simulink model "DFIG_FILTER"  (R2023a)
settings: Solver=ode23t  StartTime=0.0  StopTime=25  MaxStep=1e-6  RelTol=1e-3
model workspace (MAT data in the model file):
  Ts_phasor = 10
undefined symbols (not defined in the file): Base_Power, D1, Delta, F, find_system, Fnom, gcbh, H, ILd_init, ILq_init, Imax_grid_conv, Init, j, Ki_dc_reg, Ki_grid_side_cur_reg, Ki_power_reg, Ki_Q, Ki_rotor_side_cur_reg, Ki_volt_reg, Kp_dc_reg, Kp_grid_side_cur_reg, Kp_power_reg, Kp_Q, Kp_rotor_side_cur_reg, Kp_volt_reg, L_RL, Llr, Lls, p, Pnom, power_A, power_B, power_D, R_RL, Rr, Rs, speed_A, speed_B, speed_C, speed_D, sps_rtmsupport, Vcontrol, Vnom, Wind_On
libraries: spsPower3phPhasorLib x9, spsOnDelayLib x9, spsThreePhaseVIMeasurementLib x8, simulink_extras x5, spsRMSLib x4, spsControlledCurrentSourceLib x4, spsGroundLib x3, spsSeriesRLCBranchLib x2, spsThreePhaseSeriesRLCBranchLib x2, spspowerguiLib x2, spsThreePhasePISectionLineLib x2, spsThreePhaseTransformerTwoWindingsLib x2
(part 1 of 6)
settings Model: Creator=Production  LastModifiedBy=Adham
settings SolverCC: ZeroCrossAlgorithm=Adaptive
settings DebuggingCC: IgnoredZcDiagnostic=none

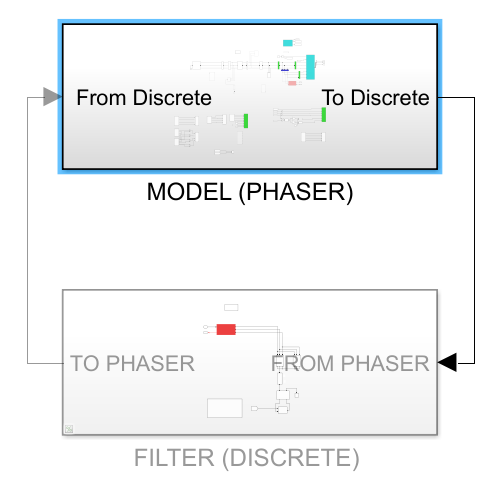
[thumbnail: Simulink's stored preview of the top-level diagram]
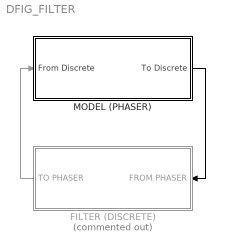
== system DFIG_FILTER ==
  "FILTER (DISCRETE) " : Subsystem  Commented=on
  MODEL (PHASER) : Subsystem
  wires:
  "FILTER (DISCRETE) "/1(TO PHASER) -> MODEL (PHASER)/1(" From Discrete")
  MODEL (PHASER)/1(To Discrete) -> "FILTER (DISCRETE) "/1(FROM PHASER)

== system DFIG_FILTER/FILTER (DISCRETE)  ==
  note: Rf
  note: Lf
  FROM PHASER : Inport
  " 1" : spsSeriesRLCBranchLib/Series RLC Branch  LConnTagsString=__new0  RConnTagsString=__new0  BranchType=RL  Resistance=0.15  Inductance=3e-3  SetiL0=off  InitialCurrent=0  Capacitance=1e-6  Setx0=off  InitialVoltage=0  Measurements=None
  CF : spsThreePhaseSeriesRLCBranchLib/Three-Phase Series RLC Branch  LConnTagsString=A|B|C  RConnTagsString=A|B|C  BranchType=C  Resistance=1  Inductance=1e-3  Capacitance=275e-6  Measurements=None
  D : spsUniversalBridgeLib/Universal Bridge  Arms=2  SnubberResistance=1e5  SnubberCapacitance=inf  Device=Diodes  Ron=10e-3  Lon=0  ForwardVoltages="[  0  0  ]"  ForwardVoltage=0  GTOparameters=[ 10e-6 , 20e-6 ]  IGBTparameters=[ 1e-6 , 2e-6 ]  Measurements=None  Measurements_2=None  converterType=Rectifier
  Discrete-to-Phasor Interface1 : spsDiscreteToPhasorInterfaceLib/Discrete-to-Phasor Interface  Rc=100  F=60  Ts_phasor=50e-6
      settings: LibrarySourceBlock=sps_lib/Utilities/Discrete-to-Phasor Interface
  Ground2 : spsGroundLib/Ground  LConnTagsString=a
  IGBT Switch Sa : spsIdealSwitchLib/Ideal Switch  Ron=0.001  Lon=0  IC=0  Rs=1e5  Cs=inf  Measurements=off
  RD : spsThreePhaseSeriesRLCBranchLib/Three-Phase Series RLC Branch  LConnTagsString=A|B|C  RConnTagsString=A|B|C  BranchType=R  Resistance=1e6  Inductance=23e-3  Capacitance=1e-6  Measurements=None
  controller1 : Subsystem
  powergui : spspowerguiLib/powergui  Priority=1  SimulationMode=Discrete  SampleTime=50e-6  frequency=60  Iterations=50  frequencyindice=0  Pbase=100e6  ErrMax=1e-4  UnitsV=kV  UnitsW=MW  buscounter=0  FunctionMessages=off  echomessages=off  EnableUseOfTLC=off  CurrentSourceSwitches=off  DisableSnubberDevices=off  DisableRonSwitches=off  DisableVfSwitches=off  DisplayEquations=off  AutomaticDiscreteSolvers=off  SolverType=Tustin/Backward Euler (TBE)  Interpol=off  ExternalGateDelay=off  methode=off  Ts=100  x0status=blocks  SPID=on  SwTol=0  HookPort=off  NonlinearTolerance=1e-4  nMaxIteration=100  ContinueOnMaxIteration=off  RestoreLinks=warning  ResistiveCurrentMeasurement=off  Frange=[0:2:500]  Ylog=off  Xlog=on  ShowGrid=off  save=off  variable=ZData  structure=0  ZoomFFT=off  StartTime=0.0  cycles=1  DisplayStyle=1  fundamental=60  FreqAxis=off  MaxFrequency=1000  frequencyindicesteady=1  RmsSteady=1  display=off
  TO PHASER : Outport
  wires:
  Discrete-to-Phasor Interface1/1 -> TO PHASER/1
  FROM PHASER/1 -> Discrete-to-Phasor Interface1/1
  [Sa] -> IGBT Switch Sa/1
  connections:
  RD/LConn3 -- Discrete-to-Phasor Interface1/LConn3 -- CF/LConn3
  RD/RConn1 -- CF/RConn3 -- CF/RConn1 -- RD/RConn3 -- RD/RConn2
  CF/RConn2 -- " 1"/LConn1
  IGBT Switch Sa/RConn1 -- D/RConn2
  " 1"/RConn1 -- D/LConn1
  IGBT Switch Sa/LConn1 -- D/RConn1
  D/LConn2 -- Ground2/LConn1
  RD/LConn2 -- Discrete-to-Phasor Interface1/LConn2 -- CF/LConn2
  CF/LConn1 -- Discrete-to-Phasor Interface1/LConn1 -- RD/LConn1

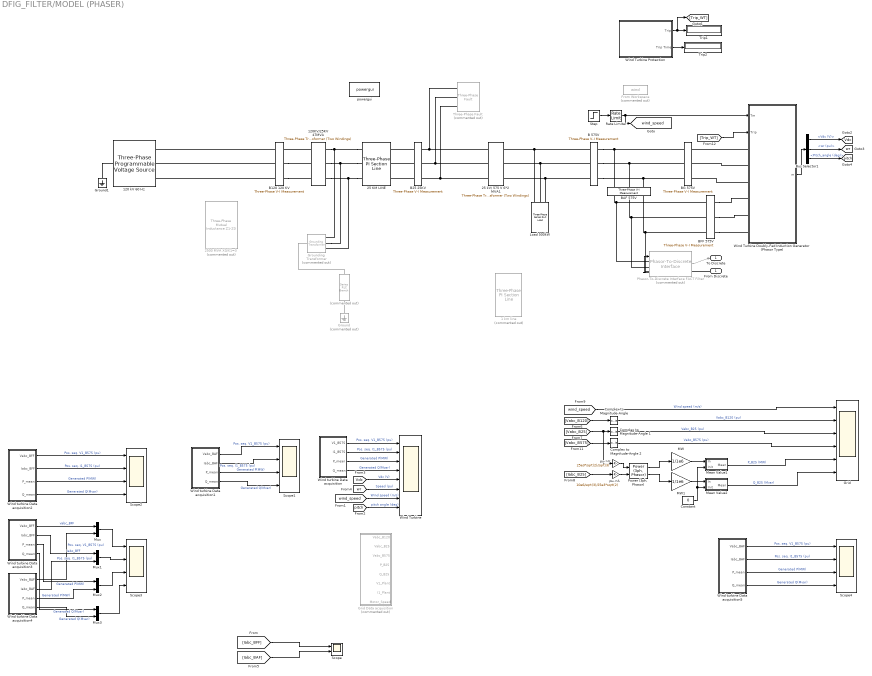
== system DFIG_FILTER/MODEL (PHASER) ==
  " From Discrete" : Inport
  " " : spsSeriesRLCBranchLib/Series RLC Branch  Commented=on  LConnTagsString=__new0  RConnTagsString=__new0  BranchType=R  Resistance=3.3  Inductance=0.003  SetiL0=off  InitialCurrent=0  Capacitance=1e-6  Setx0=off  InitialVoltage=0  Measurements=Branch voltage and current
  1 km line : spsThreePhasePISectionLineLib/Three-Phase PI Section Line  Commented=on  LConnTagsString=a|b|c  RConnTagsString=A|B|C  Length=1  Frequency=60  Resistances=[0.1153 0.413]  Inductances=[1.05e-3 3.32e-3]  Capacitances=[11.33e-009 5.01e-009]
  120 kV 60 Hz : spsThreePhaseProgrammableVoltageSourceLib/Three-Phase Programmable Voltage Source  PositiveSequence=[120e3 0 60]  VariationEntity=None  VariationType=Table of time-amplitude pairs  VariationTypeAlt=Step  VariationStep=0.5  VariationRate=10  VariationMagnitude=0.3  VariationFrequency=2  VariationTiming=[1 2]  VariationPhaseA=off  Amplitudes=[1 0.8 1.2 1.0]  TimeValues=[0 0.1 0.15 0.2]  HarmonicGeneration=off  HarmonicA=[3 0.2 -25 0]  HarmonicB=[2 0.15 35 2]  Timing="[0.05  3]"  BusType=swing  Pref=0  Qref=0  Qmin=-inf  Qmax=inf
  120KV/25KV 47MVA : spsThreePhaseTransformerTwoWindingsLib/Three-Phase Transformer (Two Windings)  Winding1Connection=Yg  Winding2Connection=Delta (D1)  CoreType=Three single-phase transformers  SetSaturation=off  Hysteresis=off  DataFile='hysteresis'  SetInitialFlux=off  Measurements=None  UNITS=pu  NominalPower=[47e6 60 ]  Winding1="[ 120e3  0.08/30   0.08 ]"  Winding2="[ 25e3  0.08/30  0.08]"  Rm=500/((120e3)^2/(Base_Power))  Lm=500/((120e3)^2/(Base_Power))  L0=0.5  Saturation=[ 0,0 ; 0.0024,1.2 ; 1.0,1.52 ]  InitialFluxes=[ 0.8 , -0.8 , 0.7 ]  BreakLoop=off  DiscreteSolver=Trapezoidal iterative  DataType=off  TransfoNumber=1
  25 KM LINE : spsThreePhasePISectionLineLib/Three-Phase PI Section Line  LConnTagsString=a|b|c  RConnTagsString=A|B|C  Length=25  Frequency=60  Resistances=[0.1153 0.413]  Inductances=[1.05e-3 3.32e-3]  Capacitances=[11.33e-009 5.01e-009]
  25 kV/ 575 V 6*2 MVA1 : spsThreePhaseTransformerTwoWindingsLib/Three-Phase Transformer (Two Windings)  Winding1Connection=Yg  Winding2Connection=Delta (D1)  CoreType=Three single-phase transformers  SetSaturation=off  Hysteresis=off  DataFile='hysteresis'  SetInitialFlux=off  Measurements=None  UNITS=pu  NominalPower="[2e6*6  60]"  Winding1=[25e3 , 0.025/30 , 0.025]  Winding2=[575, 0.025/30 , 0.025]  Rm=500/((25e3)^2/(Base_Power))  Lm=500/((25e3)^2/(Base_Power))  L0=0.5  Saturation=[ 0,0 ; 0.0024,1.2 ; 1.0,1.52 ]  InitialFluxes=[ 0.8 , -0.8 , 0.7 ]  BreakLoop=off  DiscreteSolver=Trapezoidal iterative  DataType=off  TransfoNumber=0
  2500 MVA X0/X1=3 : spsThreePhaseMutualInductanceZ1Z0Lib/Three-Phase Mutual Inductance Z1-Z0  Commented=on  LConnTagsString=a|b|c  RConnTagsString=A|B|C  PositiveSequence="[0.1  1.0/(2*pi*60)] *120e3^2/2500e6"  ZeroSequence="[0.3  3.0/(2*pi*60)] *120e3^2/2500e6"
      settings: AttributesFormatString=\n
      settings: LibrarySourceBlock=|
      | sps_lib/Power Grid Elements/Three-Phase
      | Mutual Inductance
      | Z1-Z0
  B 575V : spsThreePhaseVIMeasurementLib/Three-Phase V-I Measurement  VoltageMeasurement=phase-to-ground  SetLabelV=on  LabelV=Vabc_B575  Vpu=on  VpuLL=off  CurrentMeasurement=yes  SetLabelI=on  LabelI=Iabc_BL  Ipu=on  Pbase=Base_Power  Vbase=575  OutputType=Magnitude  PhasorSimulation=on  PSBequivalent=0
  B120 120 KV : spsThreePhaseVIMeasurementLib/Three-Phase V-I Measurement  VoltageMeasurement=phase-to-ground  SetLabelV=on  LabelV=Vabc_B120  Vpu=on  VpuLL=off  CurrentMeasurement=no  SetLabelI=on  LabelI=Iabc  Ipu=on  Pbase=100e6  Vbase=120e3  OutputType=Complex  PhasorSimulation=on  PSBequivalent=0
  B25 25KV : spsThreePhaseVIMeasurementLib/Three-Phase V-I Measurement  VoltageMeasurement=phase-to-ground  SetLabelV=on  LabelV=Vabc_B25  Vpu=on  VpuLL=off  CurrentMeasurement=yes  SetLabelI=on  LabelI=Iabc_B25  Ipu=on  Pbase=Base_Power  Vbase=25e3  OutputType=Complex  PhasorSimulation=on  PSBequivalent=0
  BAF 575V : spsThreePhaseVIMeasurementLib/Three-Phase V-I Measurement  VoltageMeasurement=phase-to-ground  SetLabelV=on  LabelV=Vabc_BAF  Vpu=on  VpuLL=off  CurrentMeasurement=yes  SetLabelI=on  LabelI=Iabc_BAF  Ipu=on  Pbase=100e6  Vbase=575  OutputType=Magnitude  PhasorSimulation=on  PSBequivalent=0
  BFF 575V : spsThreePhaseVIMeasurementLib/Three-Phase V-I Measurement  VoltageMeasurement=phase-to-ground  SetLabelV=on  LabelV=Vabc_BFF  Vpu=on  VpuLL=off  CurrentMeasurement=yes  SetLabelI=on  LabelI=Iabc_BFF  Ipu=on  Pbase=Base_Power  Vbase=575  OutputType=Magnitude  PhasorSimulation=on  PSBequivalent=0
  "BG 575V " : spsThreePhaseVIMeasurementLib/Three-Phase V-I Measurement  VoltageMeasurement=phase-to-ground  SetLabelV=on  LabelV=Vabc_BG  Vpu=on  VpuLL=off  CurrentMeasurement=yes  SetLabelI=on  LabelI=Iabc_BG  Ipu=on  Pbase=Base_Power  Vbase=575  OutputType=Complex  PhasorSimulation=on  PSBequivalent=0
  Bus Selector1 : BusSelector  OutputSignals=Vdc (V),wr (pu),Pitch_angle (deg)
  "Complex to Magnitude-Angle " : ComplexToMagnitudeAngle  Output=Magnitude
  Complex to Magnitude-Angle 1 : ComplexToMagnitudeAngle  Output=Magnitude
  Complex to Magnitude-Angle 2 : ComplexToMagnitudeAngle  Output=Magnitude
  Constant : Constant  Value=0
  From Workspace : FromWorkspace  Commented=on  VariableName=wind
  Grid : Scope  NumInputPorts=6
  Grid Data acquisition : Subsystem  Commented=on
  Ground : spsGroundLib/Ground  Commented=on  LConnTagsString=a
  Ground1 : spsGroundLib/Ground  LConnTagsString=a
  "Grounding Transformer " : spsGroundingTransformerLib/Grounding Transformer   Commented=on  UNITS=pu  NominalPower="[100e6   60]"  NominalVoltage=25e3  ZeroSequenceImpedance_pu=[0.025 0.75]  MagnetizationBranch_pu=[500 500]  ZeroSequenceImpedance_SI=[0.052083 589.05]  MagnetizationBranch_SI=[1041.7 3.927e+005]  Measurements=None
  Load 500kW : spsThreePhaseSeriesRLCLoadLib/Three-Phase Series RLC Load  LConnTagsString=A|B|C  Configuration=Y (grounded)  NominalVoltage=575  Vabc=[1e3 1e3 1e3]  Vabcp=[1e3 1e3 1e3]  NominalFrequency=60  UnbalancedPower=off  ActivePower=500e3  InductivePower=0  CapacitivePower=0  Pabc=[10e3 9e3 11e3]  QLabc=[100 90 110]  QCabc=[100 90 110]  Pabcp=[10e3 9e3 11e3]  QLabcp=[100 90 110]  QCabcp=[100 90 110]  Measurements=None  LoadType=constant Z
  MW : Gain  Gain=1/1e6  SaturateOnIntegerOverflow=on  OutDataTypeStr=Inherit: Same as input  ParamDataTypeStr=Inherit: Same as input
  MW1 : Gain  Gain=1/1e6  SaturateOnIntegerOverflow=on  OutDataTypeStr=Inherit: Same as input  ParamDataTypeStr=Inherit: Same as input
  Mean Value1 : Subsystem  mask(Mean value){Period=1/60}
      mask prompts: Period "Averaging period (s):"
      mask help: This block uses the running window averaging technique to compute the mean value of the input signal over the specified period.
  Mean Value2 : Subsystem  mask(Mean value){Period=1/60}
      mask prompts: Period "Averaging period (s):"
      mask help: This block uses the running window averaging technique to compute the mean value of the input signal over the specified period.
  Mux{,1..3} (4 alike) : Mux  Inputs=2
  Phasor-To-Discrete Interface FACT Filter : spsPhasorToDiscreteInterfaceLib/Phasor-To-Discrete Interface  Commented=on  Rc=100  F=60  Ts=50e-6
      settings: LibrarySourceBlock=sps_lib/Utilities/Phasor-To-Discrete Interface
  "Power (3ph, Phasor)" : spsPower3phPhasorLib/Power (3ph, Phasor)
  Rate Limiter : RateLimiter
  Scope : Scope  NumInputPorts=2
  Scope{1..4} (4 alike) : Scope  NumInputPorts=4
  Step : Step  Time=2  Before=4  After=14  SampleTime=0
  Three-Phase Fault : spsThreePhaseFaultLib/Three-Phase Fault  Commented=on  InitialStates=0  FaultA=on  FaultB=off  FaultC=off  GroundFault=on  SwitchTimes="[1/60  5/60]"  External=off  SwitchStatus=NaN  FaultResistance=0.001  GroundResistance=0.01  SnubberResistance=1e4  SnubberCapacitance=inf  Measurements=None
  Trip1 : Display
  Trip2 : Display
  Wind Turbine : Scope  NumInputPorts=8
  Wind Turbine Doubly-Fed Induction Generator (Phasor Type) : Subsystem  AncestorBlock=|  DialogController=POWERSYS.PowerSysDialog  LoadFcn=sps_rtmsupport('LoadFcn',gcbh); %find_system(gcs,'FollowLinks', 'on', 'LookUnderMasks', 'all');  StartFcn=sps_rtmsupport('StartFcn',gcbh);  StopFcn=sps_rtmsupport('StopFcn',gcbh);  mask(Wind Turbine Doubly-Fed Induction Generator (Phasor Type)){ExternalTm=off, nom=[1.5e6/0.9 575 60], sta=[ 0.00706 0.171], rot=[ 0.005 0.156], Lm=2.90, mec=[5.04 0.01 3], init=[0.2 0 0 0 0 0], speed_power=[0 0; 0.24 0.007; 0.36 0.024; 0.6 0.112; 0.96 0.46; 1.2 0.898; 1.5 0.898], Pmec=1.5e6, speed_ABCD=[0.7 0.71 1.2 1.21], power_C=0.73, wind_point_C=12, pitch_gain=500, pitch_max=45, pitch_rate=2, Pmax=0.5, Lchoke=[0.15 0.15/100], init_inductor=[0 90], Vdc_nom=1200, capacitor=10000e-6, ControlVQ=Voltage regulation, Vref=1.0, ExternalVref=off, Qref=0, ExternalQref=on, Iq_ref=0, ExternalIqref=off, Kpi_volt_reg=[1.25 300], Xs=0.02, Kpi_Q=[0.05 5], Kpi_power_reg=[1 100], Kpi_dc_reg=[0.002 0.05], Kpi_grid_side_cur_reg=[1 100], Kpi_rotor_side_cur_reg=[0.3 8], V_slew_rate=100, Q_slew_rate=100, power_slew_rate=1, current_slew_rate=200}
      | sps_lib/Electrical Machines/Wind Turbine
      | Doubly-Fed Induction Generator
      | (Phasor Type)
      mask prompts: ExternalTm "External turbine (Tm mechanical torque input)"; nom "Nominal power, line-to-line voltage, frequency [Pn(VA), Vn(Vrms), fn(Hz)]:"; sta "Stator [Rs, Lls] (pu):"; rot "Rotor [Rr', Llr' ] (pu):"; Lm "Magnetizing inductance Lm (pu):"; mec "Inertia constant, friction factor, and pairs of poles [H(s), F(pu),  p ]:"; init "Initial conditions [s,  th(deg),  Is(pu), ph_Is(deg),  Ir(pu),  ph_Ir(deg)]:"; speed_power "Electric power-speed characteristic: [wr1(pu) p1(pu); wr2(pu) p2(pu); ... ]"; Pmec "Nominal wind turbine mechanical output power (W):"; speed_ABCD "Tracking characteristic speeds: [speed_A(pu) ... speed_D(pu)]"; power_C "Power at point C (pu/mechanical power):"; wind_point_C "Wind speed at point C (m/s):"; pitch_gain "Pitch angle controller gain [Kp]:"; pitch_max "Maximum pitch angle (deg):"; pitch_rate "Maximum rate of change of pitch angle (deg/s):"; Pmax "Converter maximum power (pu):"; Lchoke "Grid-side coupling inductor [L (pu) R (pu)]:"; init_inductor "Coupling inductor initial current: [ IL(pu) ph_IL(deg)]"; Vdc_nom "Nominal DC bus voltage (V):"; capacitor "DC bus capacitor (F):"; ControlVQ "Mode:"; Vref "Reference grid voltage Vref (pu):"; ExternalVref "External"; Qref "Generated reactive power Qref (pu):"; ExternalQref "External"; Iq_ref "Grid-side converter generated reactive current reference (Iq_ref) (pu):"; ExternalIqref "External"; Kpi_volt_reg "Grid voltage regulator gains: [Kp Ki]"; Xs "Droop Xs (pu):"; Kpi_Q "Reactive power regulator gains: [Kp Ki]"; Kpi_power_reg "Power regulator gains: [Kp Ki]"; Kpi_dc_reg "DC bus voltage regulator gains: [Kp Ki]"; Kpi_grid_side_cur_reg "Grid-side converter current regulator gains: [Kp Ki]"; Kpi_rotor_side_cur_reg "Rotor-side converter current regulator gains: [Kp Ki]"; V_slew_rate "Maximum rate of change of reference grid voltage (pu/s):"; Q_slew_rate "Maximum rate of change of reference reactive power (pu/s):"; power_slew_rate "Maximum rate of change of reference power (pu/s):"; current_slew_rate "Maximum rate of change of converter  reference currents (pu/s):"
      mask help: Implements a phasor model of a doubly-fed induction generator driven by a wind turbine.
      mask init:
      | [Pnom,Vnom,Fnom,Rs,Lls,Rr,Llr,H,p,F,Wind_On,FACTSroot,mag_IL_init,ph_IL_init,ILd_init,ILq_init,Imax_grid_conv,speed_A,speed_B,speed_C,speed_D,power_A,power_B,power_D,L_RL,R_RL,Kp_volt_reg,Ki_volt_reg,Kp_Q,Ki_Q,Kp_power_reg,Ki_power_reg,Kp_dc_reg,Ki_dc_reg,Kp_grid_side_cur_reg,Ki_grid_side_cur_reg,Kp_rotor_side_cur_reg,Ki_rotor_side_cur_reg,Vcontrol] ...
      |     = WindTurbineInit (nom,sta,rot,mec,ExternalTm,1,gcbh,Pmax,Lchoke,init_inductor,speed_ABCD,power_C,Kpi_volt_reg,Kpi_Q,Kpi_power_reg,Kpi_dc_reg,Kpi_grid_side_cur_reg,Kpi_rotor_side_cur_reg,ControlVQ);
      settings: CopyFcn=sps_rtmsupport('CopyFcn',gcbh);  DeleteFcn=sps_rtmsupport('DeleteFcn',gcbh);  UndoDeleteFcn=sps_rtmsupport('UndoDeleteFcn',gcbh);  ModelCloseFcn=sps_rtmsupport('ModelCloseFcn',gcbh);  PreSaveFcn=sps_rtmsupport('PreSaveFcn',gcbh);  PostSaveFcn=sps_rtmsupport('PostSaveFcn',gcbh);  NameChangeFcn=sps_rtmsupport('NameChangeFcn',gcbh);  PreCopyFcn=sps_rtmsupport('PreCopyFcn',gcbh);  OpenFcn=sps_rtmsupport('OpenFcn',gcbh, [1 21,23,25,27]);  CloseFcn=sps_rtmsupport('CloseFcn',gcbh);  PreDeleteFcn=sps_rtmsupport('PreDeleteFcn',gcbh);
      settings: LibrarySourceBlock=|
      | sps_lib/Electrical Machines/Wind Turbine
      | Doubly-Fed Induction Generator
      | (Phasor Type)
      mask Help: helpview(psbhelp)
      mask Callback ExternalTm: WindTurbineCback(gcbh);
      mask TypeOptions ControlVQ: Voltage regulation | Var regulation
      mask Callback ControlVQ: WindTurbineCback(gcbh);
      mask Callback ExternalVref: WindTurbineCback(gcbh);
      mask Callback ExternalQref: WindTurbineCback(gcbh);
      mask Callback ExternalIqref: WindTurbineCback(gcbh);
      mask DialogControl generatordata Prompt: Generator
      mask DialogControl turbinedata Prompt: Turbine
      mask DialogControl Display Prompt: Display wind turbine power characteristics
      mask DialogControl Display Callback: WindTurbineDisplay(gcbh);
      mask DialogControl convertersdata Prompt: Converters
      mask DialogControl controlparameters Prompt: Control
      mask Display:
      | port_label('LConn',1,'A_stator')
      | port_label('LConn',2,'B_stator')
      | port_label('LConn',3,'C_stator')
      | port_label('LConn',4,'A_rotor')
      | port_label('LConn',5,'B_rotor')
      | port_label('LConn',6,'C_rotor')
      | 
      | port_label('output',1,'m')
      | 
      | Block = gcbh;
      | switch get_param(Block,'ExternalTm')
      |     case 'on'
      |         port_label('input',1,'Tm')
      |     case 'off'
      |         port_label('input',1,'wind')
      | end
      | 
      | x = 2;
      | 
      | switch get_param(Block,'ControlVQ')
      |     case 'Voltage regulation'
      |         switch get_param(Block,'ExternalVref')
      |             case 'on'
      |                 port_label('input',2,'Vref');
      |                 x = 3;
      |         end
      |     case 'Var regulation'
      |         switch get_param(Block,'ExternalQref')
      |             case 'on'
      |                 port_label('input',2,'Qref');
      |                 x = 3;
      |         end
      | end
      | 
      | switch get_param(Block,'ExternalIqref')
      |     case 'on'
      |         port_label('input',x,'Iq_ref');
      |         x = x +1;
      | end
      | 
      | port_label('input',x,'trip');
  Wind Turbine Protection : Subsystem
      mask Display: disp('Wind\nTurbine\nProtection')
  Wind turbine Data acquisition : Subsystem
  Wind turbine Data acquisition1 : Subsystem
  Wind turbine Data acquisition2 : Subsystem
  Wind turbine Data acquisition3 : Subsystem
  Wind turbine Data acquisition4 : Subsystem
  Wind turbine Data acquisition5 : Subsystem
  powergui : spspowerguiLib/powergui  Priority=1  SimulationMode=Discrete phasor  SampleTime=5e-6  frequency=60  Iterations=50  frequencyindice=60  Pbase=100e6  ErrMax=1e-4  UnitsV=kV  UnitsW=MW  buscounter=0  FunctionMessages=off  echomessages=off  EnableUseOfTLC=off  CurrentSourceSwitches=off  DisableSnubberDevices=off  DisableRonSwitches=off  DisableVfSwitches=off  DisplayEquations=off  AutomaticDiscreteSolvers=off  SolverType=Tustin/Backward Euler (TBE)  Interpol=off  ExternalGateDelay=off  methode=off  Ts=100  x0status=blocks  SPID=on  SwTol=0  HookPort=off  NonlinearTolerance=1e-4  nMaxIteration=100  ContinueOnMaxIteration=off  RestoreLinks=warning  ResistiveCurrentMeasurement=off  Frange=[0:2:500]  Ylog=off  Xlog=on  ShowGrid=off  save=off  variable=ZData  structure=0  ZoomFFT=off  StartTime=0.0  cycles=1  DisplayStyle=1  fundamental=60  FreqAxis=off  MaxFrequency=1000  frequencyindicesteady=1  RmsSteady=1  display=off
  pu->A : Gain  Gain=10e6/sqrt(3)/25e3*sqrt(2)  SaturateOnIntegerOverflow=on  OutDataTypeStr=Inherit: Same as input  ParamDataTypeStr=Inherit: Same as input
  pu->V : Gain  Gain=25e3*sqrt(2)/sqrt(3)  SaturateOnIntegerOverflow=on  OutDataTypeStr=Inherit: Same as input  ParamDataTypeStr=Inherit: Same as input
  To Discrete : Outport
  tag scope: Vdc=global, pitch=global, wind_speed=global, wr=global
  wires:
  [Trip_WT] -> Wind Turbine Doubly-Fed Induction Generator (Phasor Type)/2(Trip)
  Bus Selector1/3 -> [pitch]  "<Pitch_angle (deg)>"
  Bus Selector1/1 -> [Vdc]  "<Vdc (V)>"
  Wind Turbine Doubly-Fed Induction Generator (Phasor Type)/1(m) -> Bus Selector1/1
  " From Discrete"/1 -> Phasor-To-Discrete Interface FACT Filter/1
  Bus Selector1/2 -> [wr]  "<wr (pu)>"
  Phasor-To-Discrete Interface FACT Filter/1 -> To Discrete/1
  Wind turbine Data acquisition/4(Q_mean) -> Wind Turbine/4  "Generated Q(Mvar)"
  [wind_speed] -> Wind Turbine/7  "Wind speed (m/s)"
  Complex to Magnitude-Angle 2/1 -> Grid/4  "Vabc_B575 (pu)"
  Wind turbine Data acquisition/2(I1_B575) -> Wind Turbine/2  "Pos. seq. I1_B575 (pu)"
  Mean Value1/1(Mean) -> Grid/5  "P_B25 (MW)"
  Complex to Magnitude-Angle 1/1 -> Grid/3  "Vabc_B25 (pu)"
  [wr] -> Wind Turbine/6  "Speed (pu)"
  Wind turbine Data acquisition/3(P_mean) -> Wind Turbine/3  "Generated P(MW)"
  "Complex to Magnitude-Angle "/1 -> Grid/2  "Vabc_B120 (pu)"
  [pitch] -> Wind Turbine/8  "pitch angle (deg)"
  Mean Value2/1(Mean) -> Grid/6  "Q_B25 (Mvar)"
  Wind turbine Data acquisition/1(V1_B575) -> Wind Turbine/1  "Pos. seq. V1_B575 (pu)"
  [Vdc] -> Wind Turbine/5  "Vdc (V)"
  Wind Turbine Protection/2(Trip Time) -> Trip2/1
  Wind Turbine Protection/1(Trip) -> [Trip_WT], Trip1/1
  Step/1 -> Rate Limiter/1
  Rate Limiter/1 -> [wind_speed], Wind Turbine Doubly-Fed Induction Generator (Phasor Type)/1("Tm ")
  [Iabc_BFF] -> Scope/1
  [Iabc_BAF] -> Scope/2
  Wind turbine Data acquisition1/1(Vabc_BAF) -> Scope1/1  "Pos. seq. V1_B575 (pu)"
  Wind turbine Data acquisition1/2(Iabc_BAF) -> Scope1/2  "Pos. seq. I1_B575 (pu)"
  Wind turbine Data acquisition1/3(P_mean) -> Scope1/3  "Generated P(MW)"
  Wind turbine Data acquisition1/4(Q_mean) -> Scope1/4  "Generated Q(Mvar)"
  Wind turbine Data acquisition2/2(Iabc_BFF) -> Scope2/2  "Pos. seq. I1_B575 (pu)"
  Wind turbine Data acquisition2/3(P_mean) -> Scope2/3  "Generated P(MW)"
  Wind turbine Data acquisition2/1(Vabc_BFF) -> Scope2/1  "Pos. seq. V1_B575 (pu)"
  Wind turbine Data acquisition2/4(Q_mean) -> Scope2/4  "Generated Q(Mvar)"
  Wind turbine Data acquisition3/1(Vabc_BFF) -> Mux/1  "vabc_BFF"
  Wind turbine Data acquisition4/1(Vabc_BAF) -> Mux/2  "Pos. seq. V1_B575 (pu)"
  Wind turbine Data acquisition3/2(Iabc_BFF) -> Mux1/1  "Iabc_BFF"
  Wind turbine Data acquisition4/2(Iabc_BAF) -> Mux1/2  "Pos. seq. I1_B575 (pu)"
  Wind turbine Data acquisition3/3(P_mean) -> Mux2/1  "Generated P(MW)"
  Wind turbine Data acquisition4/3(P_mean) -> Mux2/2  "Generated P(MW)"
  Wind turbine Data acquisition4/4(Q_mean) -> Mux3/2  "Generated Q(Mvar)"
  Wind turbine Data acquisition3/4(Q_mean) -> Mux3/1  "Generated Q(Mvar)"
  Mux/1 -> Scope3/1
  Mux1/1 -> Scope3/2
  Mux2/1 -> Scope3/3
  Mux3/1 -> Scope3/4
  [Vabc_B575] -> Complex to Magnitude-Angle 2/1
  [Vabc_B120] -> "Complex to Magnitude-Angle "/1
  MW/1 -> Mean Value1/1(In)
  MW1/1 -> Mean Value2/1(In)
  "Power (3ph, Phasor)"/1 -> MW/1
  pu->A/1 -> "Power (3ph, Phasor)"/2
  "Power (3ph, Phasor)"/2 -> MW1/1
  Constant/1 -> Mean Value1/2(Init), Mean Value2/2(Init)
  pu->V/1 -> "Power (3ph, Phasor)"/1
  [Iabc_B25] -> pu->A/1
  [Vabc_B25] -> Complex to Magnitude-Angle 1/1, pu->V/1
  Wind turbine Data acquisition5/3(P_mean) -> Scope4/3  "Generated P(MW)"
  Wind turbine Data acquisition5/2(Iabc_BAF) -> Scope4/2  "Pos. seq. I1_B575 (pu)"
  Wind turbine Data acquisition5/4(Q_mean) -> Scope4/4  "Generated Q(Mvar)"
  Wind turbine Data acquisition5/1(Vabc_BAF) -> Scope4/1  "Pos. seq. V1_B575 (pu)"
  [wind_speed] -> Grid/1  "Wind speed (m/s)"
  connections:
  25 KM LINE/LConn1 -- "Grounding Transformer "/LConn1 -- 120KV/25KV 47MVA/RConn1
  B25 25KV/LConn3 -- 25 KM LINE/RConn3
  25 KM LINE/LConn3 -- "Grounding Transformer "/LConn3 -- 120KV/25KV 47MVA/RConn3
  B25 25KV/RConn1 -- 25 kV/ 575 V 6*2 MVA1/LConn1 -- Three-Phase Fault/LConn1
  " "/LConn1 -- "Grounding Transformer "/RConn1
  Load 500kW/LConn1 -- B 575V/LConn1 -- 25 kV/ 575 V 6*2 MVA1/RConn1
  Ground1/LConn1 -- 120 kV 60 Hz/LConn1
  B25 25KV/RConn3 -- 25 kV/ 575 V 6*2 MVA1/LConn3 -- Three-Phase Fault/LConn3
  25 KM LINE/LConn2 -- "Grounding Transformer "/LConn2 -- 120KV/25KV 47MVA/RConn2
  B120 120 KV/LConn3 -- 120 kV 60 Hz/RConn3
  B120 120 KV/LConn2 -- 120 kV 60 Hz/RConn2
  Ground/LConn1 -- " "/RConn1
  B25 25KV/RConn2 -- 25 kV/ 575 V 6*2 MVA1/LConn2 -- Three-Phase Fault/LConn2
  B25 25KV/LConn1 -- 25 KM LINE/RConn1
  120KV/25KV 47MVA/LConn1 -- B120 120 KV/RConn1
  B120 120 KV/LConn1 -- 120 kV 60 Hz/RConn1
  B25 25KV/LConn2 -- 25 KM LINE/RConn2
  B120 120 KV/RConn3 -- 120KV/25KV 47MVA/LConn3
  B120 120 KV/RConn2 -- 120KV/25KV 47MVA/LConn2
  Load 500kW/LConn2 -- B 575V/LConn2 -- 25 kV/ 575 V 6*2 MVA1/RConn2
  BFF 575V/RConn1 -- Wind Turbine Doubly-Fed Induction Generator (Phasor Type)/LConn4
  BFF 575V/RConn2 -- Wind Turbine Doubly-Fed Induction Generator (Phasor Type)/LConn5
  BFF 575V/RConn3 -- Wind Turbine Doubly-Fed Induction Generator (Phasor Type)/LConn6
  Load 500kW/LConn3 -- B 575V/LConn3 -- 25 kV/ 575 V 6*2 MVA1/RConn3
  BFF 575V/LConn1 -- Phasor-To-Discrete Interface FACT Filter/LConn1 -- BAF 575V/RConn1
  BFF 575V/LConn2 -- Phasor-To-Discrete Interface FACT Filter/LConn2 -- BAF 575V/RConn2
  BFF 575V/LConn3 -- BAF 575V/RConn3 -- Phasor-To-Discrete Interface FACT Filter/LConn3
  Wind Turbine Doubly-Fed Induction Generator (Phasor Type)/LConn1 -- "BG 575V "/RConn1
  Wind Turbine Doubly-Fed Induction Generator (Phasor Type)/LConn2 -- "BG 575V "/RConn2
  Wind Turbine Doubly-Fed Induction Generator (Phasor Type)/LConn3 -- "BG 575V "/RConn3
  "BG 575V "/LConn3 -- B 575V/RConn3 -- BAF 575V/LConn3
  "BG 575V "/LConn2 -- B 575V/RConn2 -- BAF 575V/LConn2
  "BG 575V "/LConn1 -- B 575V/RConn1 -- BAF 575V/LConn1

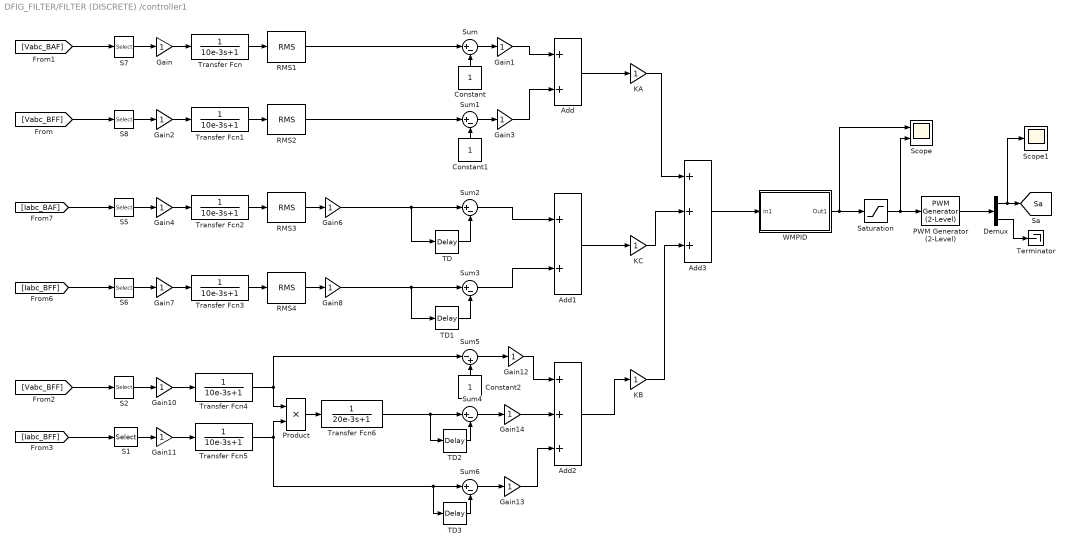
== system DFIG_FILTER/FILTER (DISCRETE) /controller1 ==
  Add : Sum
  Add1 : Sum
  Add2 : Sum  Inputs=+++
  Add3 : Sum  Inputs=+++
  Constant : Constant
  Constant1 : Constant
  Constant2 : Constant
  Demux : Demux  Outputs=2
  Gain{,1..4,6..8,10..14} (13 alike) : Gain
  KA : Gain
  KB : Gain
  KC : Gain
  PWM Generator (2-Level) : spsPWMGenerator2LevelLib/PWM Generator (2-Level)  ModulatorType=Three-phase bridge (6 pulses)  ModulatorMode=Unsynchronized  Fc=1750  Pc=90  nF=27  MinMax="[ -1  1 ]"  SamplingTechnique=Natural  ModulatingSignals=off  m=0.8  Freq=60  Phase=0  Ts=0  ShowCarrierOutport=off
  Product : Product
  RMS{1..4} (4 alike) : spsRMSLib/RMS  TrueRMS=on  Freq=60  RMSInit=120  Ts=0
  S{1..2,5..8} (6 alike) : Selector  InputPortWidth=3  IndexOptions=Index vector (dialog)  Indices=[1]  OutputSizes=1
  Saturation : Saturate  UpperLimit=1  LowerLimit=-1
  Scope : Scope  NumInputPorts=2
  Scope1 : Scope
  Sum{,1..4,6} (6 alike) : Sum  Inputs=|+-
  Sum5 : Sum  Inputs=|-+
  TD{,1..3} (4 alike) : TransportDelay  DelayTime=0.01
  Terminator : Terminator
  Transfer Fcn{,1..5} (6 alike) : TransferFcn  Denominator=[10e-3 1]
  Transfer Fcn6 : TransferFcn  Denominator=[20e-3 1]
  WMPID : Subsystem
  tag scope: Sa=global
  wires:
  [Vabc_BFF] -> S2/1
  [Iabc_BFF] -> S1/1
  Add3/1 -> WMPID/1(In1)
  Add1/1 -> KC/1
  Transfer Fcn/1 -> RMS1/1
  KA/1 -> Add3/1
  Product/1 -> Transfer Fcn6/1
  Gain14/1 -> Add2/2
  Sum6/1 -> Gain13/1
  [Vabc_BFF] -> S8/1
  Gain3/1 -> Add/2
  Sum4/1 -> Gain14/1
  Sum1/1 -> Gain3/1
  Transfer Fcn6/1 -> TD2/1, Sum4/1
  Gain8/1 -> TD1/1, Sum3/1
  [Vabc_BAF] -> S7/1
  Constant2/1 -> Sum5/2
  KB/1 -> Add3/3
  Add2/1 -> KB/1
  RMS4/1 -> Gain8/1
  Gain/1 -> Transfer Fcn/1
  [Iabc_BFF] -> S6/1
  S2/1 -> Gain10/1
  S7/1 -> Gain/1
  RMS1/1 -> Sum/1
  Transfer Fcn5/1 -> TD3/1, Sum6/1, Product/2
  [Iabc_BAF] -> S5/1
  Gain7/1 -> Transfer Fcn3/1
  Gain4/1 -> Transfer Fcn2/1
  S6/1 -> Gain7/1
  Transfer Fcn2/1 -> RMS3/1
  Constant/1 -> Sum/2
  S1/1 -> Gain11/1
  Gain2/1 -> Transfer Fcn1/1
  Constant1/1 -> Sum1/2
  Transfer Fcn3/1 -> RMS4/1
  Sum/1 -> Gain1/1
  TD3/1 -> Sum6/2
  TD1/1 -> Sum3/2
  S5/1 -> Gain4/1
  Sum2/1 -> Add1/1
  Saturation/1 -> Scope/2, PWM Generator (2-Level)/1
  Gain6/1 -> Sum2/1, TD/1
  RMS2/1 -> Sum1/1
  Transfer Fcn1/1 -> RMS2/1
  Gain1/1 -> Add/1
  Sum3/1 -> Add1/2
  KC/1 -> Add3/2
  TD2/1 -> Sum4/2
  Add/1 -> KA/1
  WMPID/1(Out1) -> Scope/1, Saturation/1
  Gain10/1 -> Transfer Fcn4/1
  S8/1 -> Gain2/1
  Sum5/1 -> Gain12/1
  RMS3/1 -> Gain6/1
  Transfer Fcn4/1 -> Sum5/1, Product/1
  Gain11/1 -> Transfer Fcn5/1
  Gain13/1 -> Add2/3
  PWM Generator (2-Level)/1 -> Demux/1
  TD/1 -> Sum2/2
  Gain12/1 -> Add2/1
  Demux/1 -> Scope1/1, [Sa]
  Demux/2 -> Terminator/1

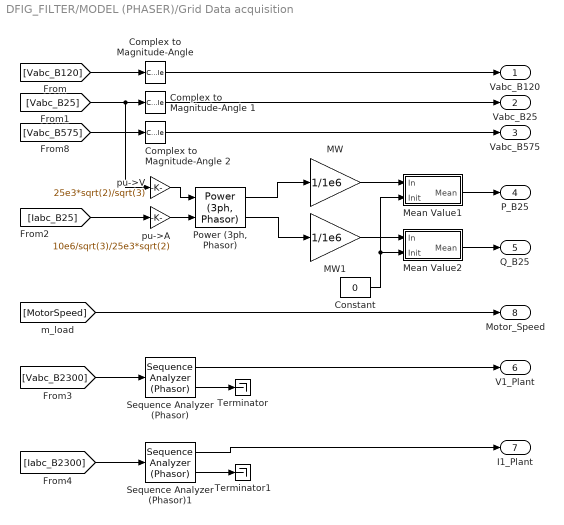
== system DFIG_FILTER/MODEL (PHASER)/Grid Data acquisition ==
  "Complex to Magnitude-Angle " : ComplexToMagnitudeAngle  Output=Magnitude
  Complex to Magnitude-Angle 1 : ComplexToMagnitudeAngle  Output=Magnitude
  Complex to Magnitude-Angle 2 : ComplexToMagnitudeAngle  Output=Magnitude
  Constant : Constant  Value=0
  MW : Gain  Gain=1/1e6  SaturateOnIntegerOverflow=on  OutDataTypeStr=Inherit: Same as input  ParamDataTypeStr=Inherit: Same as input
  MW1 : Gain  Gain=1/1e6  SaturateOnIntegerOverflow=on  OutDataTypeStr=Inherit: Same as input  ParamDataTypeStr=Inherit: Same as input
  Mean Value1 : Subsystem  mask(Mean value){Period=1/60}
      mask prompts: Period "Averaging period (s):"
      mask help: This block uses the running window averaging technique to compute the mean value of the input signal over the specified period.
  Mean Value2 : Subsystem  mask(Mean value){Period=1/60}
      mask prompts: Period "Averaging period (s):"
      mask help: This block uses the running window averaging technique to compute the mean value of the input signal over the specified period.
  "Power (3ph, Phasor)" : spsPower3phPhasorLib/Power (3ph, Phasor)
  Sequence Analyzer (Phasor) : spsSequenceAnalyzerPhasorLib/Sequence Analyzer (Phasor)  seq=Positive
  Sequence Analyzer (Phasor)1 : spsSequenceAnalyzerPhasorLib/Sequence Analyzer (Phasor)  seq=Positive
  Terminator : Terminator
  Terminator1 : Terminator
  pu->A : Gain  Gain=10e6/sqrt(3)/25e3*sqrt(2)  SaturateOnIntegerOverflow=on  OutDataTypeStr=Inherit: Same as input  ParamDataTypeStr=Inherit: Same as input
  pu->V : Gain  Gain=25e3*sqrt(2)/sqrt(3)  SaturateOnIntegerOverflow=on  OutDataTypeStr=Inherit: Same as input  ParamDataTypeStr=Inherit: Same as input
  "Vabc_B120 " : Outport  VectorParamsAs1DForOutWhenUnconnected=off
  "Vabc_B25 " : Outport  Port=2  VectorParamsAs1DForOutWhenUnconnected=off
  "Vabc_B575 " : Outport  Port=3  VectorParamsAs1DForOutWhenUnconnected=off
  P_B25 : Outport  Port=4  VectorParamsAs1DForOutWhenUnconnected=off
  Q_B25 : Outport  Port=5  VectorParamsAs1DForOutWhenUnconnected=off
  V1_Plant : Outport  Port=6  VectorParamsAs1DForOutWhenUnconnected=off
  I1_Plant : Outport  Port=7  VectorParamsAs1DForOutWhenUnconnected=off
  Motor_Speed : Outport  Port=8  VectorParamsAs1DForOutWhenUnconnected=off
  wires:
  pu->A/1 -> "Power (3ph, Phasor)"/2
  pu->V/1 -> "Power (3ph, Phasor)"/1
  "Complex to Magnitude-Angle "/1 -> "Vabc_B120 "/1
  [Vabc_B120] -> "Complex to Magnitude-Angle "/1
  Complex to Magnitude-Angle 1/1 -> "Vabc_B25 "/1
  [Vabc_B25] -> Complex to Magnitude-Angle 1/1, pu->V/1
  Complex to Magnitude-Angle 2/1 -> "Vabc_B575 "/1
  [Vabc_B575] -> Complex to Magnitude-Angle 2/1
  [Iabc_B25] -> pu->A/1
  Constant/1 -> Mean Value1/2(Init), Mean Value2/2(Init)
  Mean Value1/1(Mean) -> P_B25/1
  Mean Value2/1(Mean) -> Q_B25/1
  [MotorSpeed] -> Motor_Speed/1
  [Vabc_B2300] -> Sequence Analyzer (Phasor)/1
  Sequence Analyzer (Phasor)/1 -> V1_Plant/1
  Sequence Analyzer (Phasor)/2 -> Terminator/1
  [Iabc_B2300] -> Sequence Analyzer (Phasor)1/1
  Sequence Analyzer (Phasor)1/1 -> I1_Plant/1
  Sequence Analyzer (Phasor)1/2 -> Terminator1/1
  MW/1 -> Mean Value1/1(In)
  MW1/1 -> Mean Value2/1(In)
  "Power (3ph, Phasor)"/1 -> MW/1
  "Power (3ph, Phasor)"/2 -> MW1/1

== system DFIG_FILTER/MODEL (PHASER)/Mean Value1 ==
  note: Mean value
  In : Inport
  Init : Inport  Port=2
  Gain : Gain  Gain=1/Period  SaturateOnIntegerOverflow=on  OutDataTypeStr=Inherit: Same as input  ParamDataTypeStr=Inherit: Same as input
  Step : Step  Time=Period+eps  SampleTime=0
  Sum : Sum  Inputs=+-  InputSameDT=on  SaturateOnIntegerOverflow=on  OutDataTypeStr=Inherit: Same as first input
  Switch : Switch  Threshold=0.5  InputSameDT=off
  Transport Delay : TransportDelay  DelayTime=Period
  integrator : Integrator
  Mean : Outport  VectorParamsAs1DForOutWhenUnconnected=off
  wires:
  Transport Delay/1 -> Sum/2
  integrator/1 -> Transport Delay/1, Sum/1
  In/1 -> integrator/1
  Sum/1 -> Gain/1
  Gain/1 -> Switch/1
  Switch/1 -> Mean/1
  Step/1 -> Switch/2
  Init/1 -> Switch/3

== system DFIG_FILTER/MODEL (PHASER)/Mean Value2 ==
  note: Mean value
  In : Inport
  Init : Inport  Port=2
  Gain : Gain  Gain=1/Period  SaturateOnIntegerOverflow=on  OutDataTypeStr=Inherit: Same as input  ParamDataTypeStr=Inherit: Same as input
  Step : Step  Time=Period+eps  SampleTime=0
  Sum : Sum  Inputs=+-  InputSameDT=on  SaturateOnIntegerOverflow=on  OutDataTypeStr=Inherit: Same as first input
  Switch : Switch  Threshold=0.5  InputSameDT=off
  Transport Delay : TransportDelay  DelayTime=Period
  integrator : Integrator
  Mean : Outport  VectorParamsAs1DForOutWhenUnconnected=off
  wires:
  Init/1 -> Switch/3
  Step/1 -> Switch/2
  Switch/1 -> Mean/1
  Gain/1 -> Switch/1
  Sum/1 -> Gain/1
  In/1 -> integrator/1
  integrator/1 -> Sum/1, Transport Delay/1
  Transport Delay/1 -> Sum/2

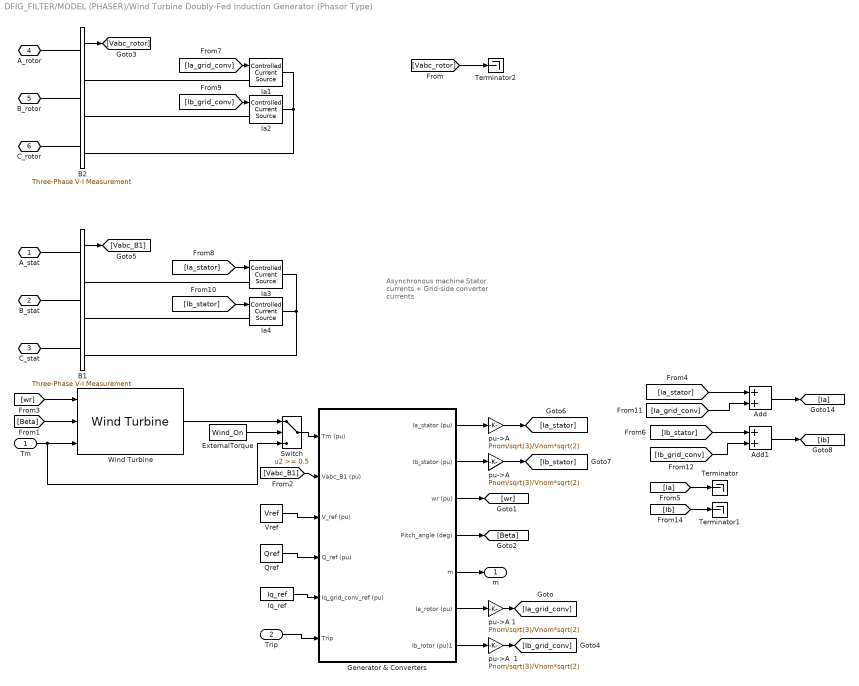
== system DFIG_FILTER/MODEL (PHASER)/Wind Turbine Doubly-Fed Induction Generator (Phasor Type) ==
  note: Asynchronous machine
      | Stator currents
      | +
      | Grid-side converter
      | currents
  "Tm " : Inport
  Trip : Inport  Port=2
  Add : Sum
  Add1 : Sum
  B1 : spsThreePhaseVIMeasurementLib/Three-Phase V-I Measurement  VoltageMeasurement=phase-to-ground  SetLabelV=off  LabelV=Vabc_B1  Vpu=on  VpuLL=off  CurrentMeasurement=no  SetLabelI=off  LabelI=Iabc_Beol  Ipu=off  Pbase=Pnom  Vbase=Vnom  OutputType=Complex  PhasorSimulation=on  PSBequivalent=0
  B2 : spsThreePhaseVIMeasurementLib/Three-Phase V-I Measurement  VoltageMeasurement=phase-to-ground  SetLabelV=off  LabelV=Vabc_B1  Vpu=on  VpuLL=off  CurrentMeasurement=no  SetLabelI=off  LabelI=Iabc_Beol  Ipu=off  Pbase=Pnom  Vbase=Vnom  OutputType=Complex  PhasorSimulation=on  PSBequivalent=0
  ExternalTorque : Constant  Value=Wind_On
  Generator & Converters : Subsystem
  Ia{1..4} (4 alike) : spsControlledCurrentSourceLib/Controlled Current Source  Description=source block  Initialize=off  Source_Type=AC  Amplitude=0  Phase=0  Frequency=0  Measurements=None
  "Iq_ref " : Constant  Value=Iq_ref
  "Qref " : Constant  Value=Qref
  Switch : Switch  Threshold=0.5  InputSameDT=off
  Terminator : Terminator
  Terminator1 : Terminator
  Terminator2 : Terminator
  "Vref " : Constant  Value=Vref
  Wind Turbine : spsWindTurbineLib/Wind Turbine  Pnom=Pmec  Pelec_base=Pnom  wind_base=wind_point_C  P_wind_base=power_C  speed_nom=speed_C  pitch_angle=0  c1_c6="[0.51763          116          0.4            5           21     0.006795]"  cp_nom=0.48  lambda_nom=8.1
  "pu->A " : Gain  Gain=Pnom/sqrt(3)/Vnom*sqrt(2)  SaturateOnIntegerOverflow=on  OutDataTypeStr=Inherit: Same as input  ParamDataTypeStr=Inherit: Same as input
  "pu->A  " : Gain  Gain=Pnom/sqrt(3)/Vnom*sqrt(2)  SaturateOnIntegerOverflow=on  OutDataTypeStr=Inherit: Same as input  ParamDataTypeStr=Inherit: Same as input
  pu->A  1 : Gain  Gain=Pnom/sqrt(3)/Vnom*sqrt(2)  SaturateOnIntegerOverflow=on  OutDataTypeStr=Inherit: Same as input  ParamDataTypeStr=Inherit: Same as input
  pu->A 1 : Gain  Gain=Pnom/sqrt(3)/Vnom*sqrt(2)  SaturateOnIntegerOverflow=on  OutDataTypeStr=Inherit: Same as input  ParamDataTypeStr=Inherit: Same as input
  A_stat : PMIOPort  Side=Left
  B_stat : PMIOPort  Port=2  Side=Left
  C_stat : PMIOPort  Port=3  Side=Left
  A_rotor : PMIOPort  Port=4  Side=Left
  B_rotor : PMIOPort  Port=5  Side=Left
  C_rotor : PMIOPort  Port=6  Side=Left
  m : Outport  VectorParamsAs1DForOutWhenUnconnected=off
  wires:
  Switch/1 -> Generator & Converters/1(Tm (pu))
  [Vabc_B1] -> Generator & Converters/2(Vabc_B1 (pu))
  Generator & Converters/1(Ia_stator (pu)) -> "pu->A "/1
  "pu->A  "/1 -> [Ib_stator]
  "pu->A "/1 -> [Ia_stator]
  B1/1 -> [Vabc_B1]
  Generator & Converters/3(wr (pu)) -> [wr]
  ExternalTorque/1 -> Switch/2
  Generator & Converters/2(Ib_stator (pu)) -> "pu->A  "/1
  "Tm "/1 -> Wind Turbine/3, Switch/3
  [wr] -> Wind Turbine/1
  Wind Turbine/1 -> Switch/1
  Generator & Converters/5(m) -> m/1
  "Qref "/1 -> Generator & Converters/4(Q_ref (pu))
  "Iq_ref "/1 -> Generator & Converters/5(Iq_grid_conv_ref (pu))
  "Vref "/1 -> Generator & Converters/3(V_ref (pu))
  [Ia_stator] -> Ia3/1
  [Ib_stator] -> Ia4/1
  Trip/1 -> Generator & Converters/6(Trip)
  [Beta] -> Wind Turbine/2
  Generator & Converters/4(Pitch_angle (deg)) -> [Beta]
  B2/1 -> [Vabc_rotor]
  [Ia_grid_conv] -> Ia1/1
  [Ib_grid_conv] -> Ia2/1
  Generator & Converters/7(Ib_rotor (pu)1) -> pu->A  1/1
  Generator & Converters/6(Ia_rotor (pu)) -> pu->A 1/1
  Add1/1 -> [Ib]
  Add/1 -> [Ia]
  pu->A 1/1 -> [Ia_grid_conv]
  pu->A  1/1 -> [Ib_grid_conv]
  [Ib_grid_conv] -> Add1/2
  [Ib_stator] -> Add1/1
  [Ia_grid_conv] -> Add/2
  [Ia_stator] -> Add/1
  [Ia] -> Terminator/1
  [Ib] -> Terminator1/1
  [Vabc_rotor] -> Terminator2/1
  connections:
  B_stat/RConn1 -- B1/LConn2
  C_stat/RConn1 -- B1/LConn3
  Ia4/LConn1 -- B1/RConn2
  A_stat/RConn1 -- B1/LConn1
  Ia3/LConn1 -- B1/RConn1
  B2/RConn2 -- Ia2/LConn1
  Ia1/LConn1 -- B2/RConn1
  B2/LConn3 -- C_rotor/RConn1
  B1/RConn3 -- Ia3/RConn1 -- Ia4/RConn1
  B2/LConn2 -- B_rotor/RConn1
  A_rotor/RConn1 -- B2/LConn1
  Ia1/RConn1 -- B2/RConn3 -- Ia2/RConn1

== system DFIG_FILTER/MODEL (PHASER)/Wind Turbine Protection ==
  note: Instantaneous AC Overcurrent
  note: AC Overcurrent (positive-sequence)
  note: AC Current Unbalance
  note: AC Undervoltage (positive-sequence)
  note: AC Overvoltage (positive-sequence)
  note: AC Voltage Unbalance (Negative-sequence)
  note: AC Voltage Unbalance (Zero-sequence)
  note: DC Overvoltage
  note: Under Speed
  note: Over Speed
  Ground2 : Ground
  Protection System : Subsystem  mask(Protection System){Freq=60, Max_Iinst=10, MaxI1=[ 1.1, 5 ], MaxI2I1=[ 0.4, 0.2], MinMaxV1=[ 0.75, 1.1, 0.1 ], MaxV2V1=[ 0.05, 0.05, 0.2 ], MaxVdc=[ 1900, 0.001 ], MaxSpeed=[ 0.3, 1.5, 5 ], Delay_Protection=5}
      mask prompts: Freq "Fundamental frequency f1 (Hz):"; Max_Iinst "Instantaneous AC Overcurrent (pu):"; MaxI1 "Maximum AC Current [ I1max(pu), Delay(s) ]:"; MaxI2I1 "Maximum AC Current Unbalance [ I2/I1max(pu), Delay(s) ]"; MinMaxV1 "AC Under/Over Voltage [ V1min(pu), V1max(pu), Delay(s) ]:"; MaxV2V1 "Maximum Voltage Unbalance [ V2/V1max(pu), V0/V1max(pu), Delay(s)]:"; MaxVdc "Maximum DC Voltage  [ Vmax(V), Delay(s) ]:"; MaxSpeed "Under/Over Speed [ Speedmin (pu), Speedmax (pu), Delay(s)]:"; Delay_Protection "Start time for protection system (s):"
      mask help:
      | Protection type:
      | 1.    Instantaneous AC Overcurrent
      | 2.    AC Overcurrent (positive-sequence)
      | 3.    AC Current Unbalance
      | 4.    AC Undervoltage (positive-sequence)
      | 5.    AC Overvoltage (positive-sequence)
      | 6.    AC Voltage Unbalance (Negative-sequence)
      | 7.    AC Voltage Unbalance (Zero-sequence)
      | 8.    DC Overvoltage
      | 9.    Under Speed
      | 10.  Over Speed
      mask init:
      | a=exp(2*pi*j/3);
      | a2=a^2;
      | Max_I1=MaxI1(1);
      | Delay_I1=MaxI1(2);
      | Max_I2_I1=MaxI2I1(1);
      | Delay_I2_I1=MaxI2I1(2);
      | Min_V1=MinMaxV1(1);
      | Max_V1=MinMaxV1(2);
      | Delay_V1=MinMaxV1(3);
      | Max_V2_V1=MaxV2V1(1);
      | Max_V0_V1=MaxV2V1(2);
      | Delay_V2_V1=MaxV2V1(3);
      | Max_Vdc=MaxVdc(1);
      | Delay_Vdc=MaxVdc(2);
      | Min_Speed=MaxSpeed(1);
      | Max_Speed=MaxSpeed(2);
      | Delay_Speed=MaxSpeed(3);
  TripData : Display
  Trip : Outport  VectorParamsAs1DForOutWhenUnconnected=off
  Trip Time : Outport  Port=2  VectorParamsAs1DForOutWhenUnconnected=off
  wires:
  Ground2/1 -> Protection System/4(Reset)
  Protection System/3(TripStatus) -> TripData/1
  [Vabc_B575] -> Protection System/1(Vabc (pu))
  [Vdc] -> Protection System/3(Vdc (V))
  [wr] -> Protection System/5(Speed (pu))
  [Iabc_B575] -> Protection System/2(Iabc (pu))
  Protection System/1(Trip) -> Trip/1
  Protection System/2(TripTime) -> Trip Time/1

== system DFIG_FILTER/MODEL (PHASER)/Wind turbine Data acquisition ==
  Constant : Constant  Value=0
  Gain3 : Gain  Gain=1/3  SaturateOnIntegerOverflow=on  OutDataTypeStr=Inherit: Same as input  ParamDataTypeStr=Inherit: Same as input
  Gain4 : Gain  Gain=1/3  SaturateOnIntegerOverflow=on  OutDataTypeStr=Inherit: Same as input  ParamDataTypeStr=Inherit: Same as input
  MW : Gain  Gain=-1/1e6  SaturateOnIntegerOverflow=on  OutDataTypeStr=Inherit: Same as input  ParamDataTypeStr=Inherit: Same as input
  MW1 : Gain  Gain=-1/1e6  SaturateOnIntegerOverflow=on  OutDataTypeStr=Inherit: Same as input  ParamDataTypeStr=Inherit: Same as input
  Mean Value1 : Subsystem  mask(Mean value){Period=1/60}
      mask prompts: Period "Averaging period (s):"
      mask help: This block uses the running window averaging technique to compute the mean value of the input signal over the specified period.
  Mean Value2 : Subsystem  mask(Mean value){Period=1/60}
      mask prompts: Period "Averaging period (s):"
      mask help: This block uses the running window averaging technique to compute the mean value of the input signal over the specified period.
  "Power (3ph, Phasor)" : spsPower3phPhasorLib/Power (3ph, Phasor)
  Sum : Sum  Inputs=1  InputSameDT=on  SaturateOnIntegerOverflow=on  OutDataTypeStr=Inherit: Same as first input
  Sum1 : Sum  Inputs=1  InputSameDT=on  SaturateOnIntegerOverflow=on  OutDataTypeStr=Inherit: Same as first input
  abc_to_pos : Gain  Gain=[1 exp(j*2*pi/3) exp(-j*2*pi/3)]  SaturateOnIntegerOverflow=on  OutDataTypeStr=Inherit: Same as input  ParamDataTypeStr=Inherit: Same as input
  abc_to_pos1 : Gain  Gain=[1 exp(j*2*pi/3) exp(-j*2*pi/3)]  SaturateOnIntegerOverflow=on  OutDataTypeStr=Inherit: Same as input  ParamDataTypeStr=Inherit: Same as input
  "magnitude positive seq. " : Subsystem
  magnitude positivie seq : Subsystem
  pu->A : Gain  Gain=(6*1.5e6/0.9)/sqrt(3)/575*sqrt(2)  SaturateOnIntegerOverflow=on  OutDataTypeStr=Inherit: Same as input  ParamDataTypeStr=Inherit: Same as input
  pu->V : Gain  Gain=575*sqrt(2)/sqrt(3)  SaturateOnIntegerOverflow=on  OutDataTypeStr=Inherit: Same as input  ParamDataTypeStr=Inherit: Same as input
  V1_B575 : Outport  VectorParamsAs1DForOutWhenUnconnected=off
  I1_B575 : Outport  Port=2  VectorParamsAs1DForOutWhenUnconnected=off
  P_mean : Outport  Port=3  VectorParamsAs1DForOutWhenUnconnected=off
  Q_mean : Outport  Port=4  VectorParamsAs1DForOutWhenUnconnected=off
  wires:
  [Iabc_BL] -> pu->A/1, abc_to_pos1/1
  [Vabc_BL] -> pu->V/1, abc_to_pos/1
  pu->A/1 -> "Power (3ph, Phasor)"/2
  pu->V/1 -> "Power (3ph, Phasor)"/1
  MW/1 -> Mean Value1/1(In)
  MW1/1 -> Mean Value2/1(In)
  "magnitude positive seq. "/1(Out1) -> I1_B575/1
  magnitude positivie seq/1(Out1) -> V1_B575/1
  abc_to_pos/1 -> Sum/1
  Sum/1 -> Gain3/1
  Sum1/1 -> Gain4/1
  Gain3/1 -> magnitude positivie seq/1(In1)
  abc_to_pos1/1 -> Sum1/1
  Gain4/1 -> "magnitude positive seq. "/1(In1)
  Mean Value1/1(Mean) -> P_mean/1
  Mean Value2/1(Mean) -> Q_mean/1
  Constant/1 -> Mean Value1/2(Init), Mean Value2/2(Init)
  "Power (3ph, Phasor)"/1 -> MW/1
  "Power (3ph, Phasor)"/2 -> MW1/1

== system DFIG_FILTER/MODEL (PHASER)/Wind turbine Data acquisition1 ==
  Constant : Constant  Value=0
  Gain3 : Gain  Gain=1/3  SaturateOnIntegerOverflow=on  OutDataTypeStr=Inherit: Same as input  ParamDataTypeStr=Inherit: Same as input
  Gain4 : Gain  Gain=1/3  SaturateOnIntegerOverflow=on  OutDataTypeStr=Inherit: Same as input  ParamDataTypeStr=Inherit: Same as input
  MW : Gain  Gain=-1/1e6  SaturateOnIntegerOverflow=on  OutDataTypeStr=Inherit: Same as input  ParamDataTypeStr=Inherit: Same as input
  MW1 : Gain  Gain=-1/1e6  SaturateOnIntegerOverflow=on  OutDataTypeStr=Inherit: Same as input  ParamDataTypeStr=Inherit: Same as input
  Mean Value1 : Subsystem  mask(Mean value){Period=1/60}
      mask prompts: Period "Averaging period (s):"
      mask help: This block uses the running window averaging technique to compute the mean value of the input signal over the specified period.
  Mean Value2 : Subsystem  mask(Mean value){Period=1/60}
      mask prompts: Period "Averaging period (s):"
      mask help: This block uses the running window averaging technique to compute the mean value of the input signal over the specified period.
  "Power (3ph, Phasor)" : spsPower3phPhasorLib/Power (3ph, Phasor)
  Sum : Sum  Inputs=1  InputSameDT=on  SaturateOnIntegerOverflow=on  OutDataTypeStr=Inherit: Same as first input
  Sum1 : Sum  Inputs=1  InputSameDT=on  SaturateOnIntegerOverflow=on  OutDataTypeStr=Inherit: Same as first input
  abc_to_pos : Gain  Gain=[1 exp(j*2*pi/3) exp(-j*2*pi/3)]  SaturateOnIntegerOverflow=on  OutDataTypeStr=Inherit: Same as input  ParamDataTypeStr=Inherit: Same as input
  abc_to_pos1 : Gain  Gain=[1 exp(j*2*pi/3) exp(-j*2*pi/3)]  SaturateOnIntegerOverflow=on  OutDataTypeStr=Inherit: Same as input  ParamDataTypeStr=Inherit: Same as input
  "magnitude positive seq. " : Subsystem
  magnitude positivie seq : Subsystem
  pu->A : Gain  Gain=(6*1.5e6/0.9)/sqrt(3)/575*sqrt(2)  SaturateOnIntegerOverflow=on  OutDataTypeStr=Inherit: Same as input  ParamDataTypeStr=Inherit: Same as input
  pu->V : Gain  Gain=575*sqrt(2)/sqrt(3)  SaturateOnIntegerOverflow=on  OutDataTypeStr=Inherit: Same as input  ParamDataTypeStr=Inherit: Same as input
  Vabc_BAF : Outport  VectorParamsAs1DForOutWhenUnconnected=off
  Iabc_BAF : Outport  Port=2  VectorParamsAs1DForOutWhenUnconnected=off
  P_mean : Outport  Port=3  VectorParamsAs1DForOutWhenUnconnected=off
  Q_mean : Outport  Port=4  VectorParamsAs1DForOutWhenUnconnected=off
  wires:
  [Iabc_BAF] -> abc_to_pos1/1, pu->A/1
  [Vabc_BAF] -> pu->V/1, abc_to_pos/1
  pu->A/1 -> "Power (3ph, Phasor)"/2
  pu->V/1 -> "Power (3ph, Phasor)"/1
  MW/1 -> Mean Value1/1(In)
  MW1/1 -> Mean Value2/1(In)
  "magnitude positive seq. "/1(Out1) -> Iabc_BAF/1
  magnitude positivie seq/1(Out1) -> Vabc_BAF/1
  abc_to_pos/1 -> Sum/1
  Sum/1 -> Gain3/1
  Sum1/1 -> Gain4/1
  Gain3/1 -> magnitude positivie seq/1(In1)
  abc_to_pos1/1 -> Sum1/1
  Gain4/1 -> "magnitude positive seq. "/1(In1)
  Mean Value1/1(Mean) -> P_mean/1
  Mean Value2/1(Mean) -> Q_mean/1
  Constant/1 -> Mean Value1/2(Init), Mean Value2/2(Init)
  "Power (3ph, Phasor)"/1 -> MW/1
  "Power (3ph, Phasor)"/2 -> MW1/1
